simulink model "model_quad_nl_mpc_nl"  (R2021b)
settings: Solver=FixedStepAuto  StartTime=0.0  StopTime=10  FixedStep=.01  MaxStep=.1  MinStep=.005  RelTol=1e-3
values from neighbouring files (symbols this model uses):
  Abody = pi*Rbody^2    (= 0.0314159265359)    [model_quad_init.m]    (also in nlStateFcn.m = 0.0314)
  CDbody = 0.75    [model_quad_init.m]    (also in nlStateFcn.m)
  CT = 0.0248    [model_quad_init.m]
  g = 9.81    [model_quad_init.m]    (also in nlStateFcn.m; nlStateFcnTest.m; start_drone.m)
  i0 = 0    [model_quad_init.m]    (also in nlStateFcn.m)
  Ibbperp = .00942    (= 0.00942)    [model_quad_init.m]    (also in nlStateFcn.m; nlStateFcnTest.m)
  Ibbxx = Ibbperp    (= 0.00942)    [model_quad_init.m]    (also in nlStateFcn.m; nlStateFcnTest.m)
  Ibbxz = 0    [model_quad_init.m]    (also in nlStateFcn.m; nlStateFcnTest.m)
  Ibbyy = Ibbperp    (= 0.00942)    [model_quad_init.m]    (also in nlStateFcn.m; nlStateFcnTest.m)
  Ibbzz = .01867    (= 0.01867)    [model_quad_init.m]    (also in nlStateFcn.m; nlStateFcnTest.m)
  Irrperp = Irrpolar/2    (= 0.0001113)    [model_quad_init.m]    (also in nlStateFcn.m; nlStateFcnTest.m)
  Irrpolar = .0002226    (= 0.0002226)    [model_quad_init.m]
  Kv = 130    [model_quad_init.m]    (also in nlStateFcn.m)
  mb = mb/m_tot    (= 0.760306807287)    [model_quad_init.m]    (also in nlStateFcn.m; nlStateFcnTest.m)
  mr = mr/m_tot    (= 0.0599232981783)    [model_quad_init.m]    (also in nlStateFcn.m; nlStateFcnTest.m)
  R_arms = .45/2    (= 0.225)    [model_quad_init.m]    (also in nlStateFcn.m; nlStateFcnTest.m)
  R_rotor = .125    (= 0.125)    [model_quad_init.m]    (also in nlStateFcn.m)
  rho = 1.225    [model_quad_init.m]    (also in nlStateFcn.m)
  rotorAero = load('loopQuadBET_fromTheBook.mat','C_T','C_H','C_M','C_Q','mu_z_loops','mu_x_loops')    [model_quad_init.m]    (also in nlStateFcn.m)
  Rwinding = 0.56    [model_quad_init.m]
  spin_dir = [1 -1 1 -1]    [model_quad_init.m]    (also in nlStateFcn.m = [1,-1,1,-1])
  Vmax = 4*3.7    (= 14.8)    [model_quad_init.m]
  z_rotors = 0    [model_quad_init.m]    (also in nlStateFcn.m; nlStateFcnTest.m)
undefined symbols (not defined in the file or in its folder): R_RB
libraries: dspmathops x1, mpclib x1
(part 1 of 2)
settings Model: Creator=Elena  LastModifiedBy=Elena

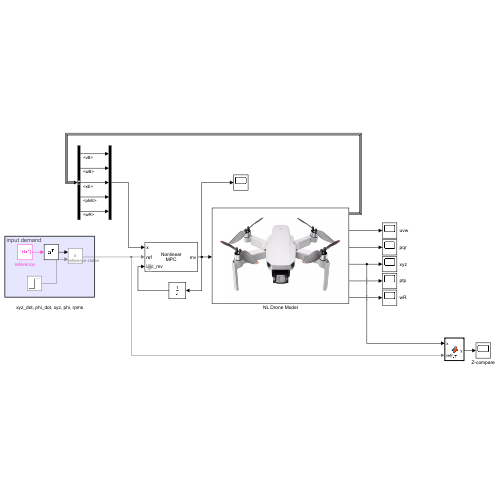
[thumbnail: Simulink's stored preview of the top-level diagram]
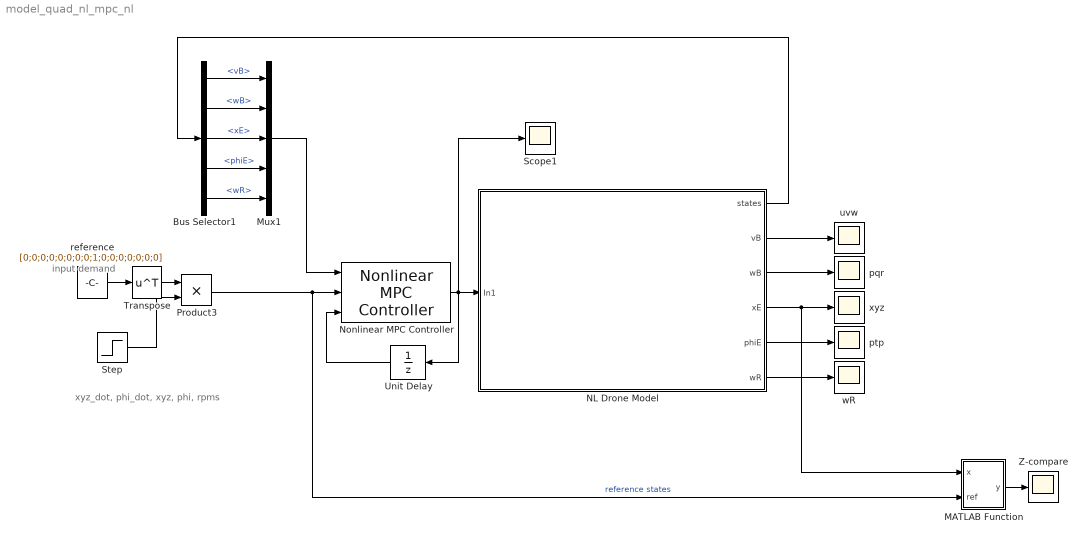
== system model_quad_nl_mpc_nl ==
  note: input demand
  note: xyz_dot, phi_dot, xyz, phi, rpms
  Bus Selector1 : BusSelector  OutputSignals=vB,wB,xE,phiE,wR
  MATLAB Function : MATLAB Function  TreatAsAtomicUnit=on
  Mux1 : Mux  Inputs=5
  NL Drone Model : Subsystem
      mask Display: image('drone_model.png'); % Use "Edit Image" on toolstrip to change.
  Nonlinear MPC Controller : mpclib/Nonlinear MPC Controller  nlmpcobj=nlobj  UseObjectTs=on  UseMEX=off  md_enabled=off  mvtarget_enabled=off  param_enabled=off  cost_enabled=off  mvseq_enabled=off  stateseq_enabled=off  ovseq_enabled=off  slack_enabled=off  status_enabled=off  ov_min=off  ov_max=off  mv_min=off  mv_max=off  mvrate_min=off  mvrate_max=off  state_min=off  state_max=off  ov_weight=off  mv_weight=off  mvrate_weight=off  ecr_weight=off  nlp_initialize=off
  Product3 : Product
  Scope1 : Scope
  Step : Step  SampleTime=0
  Transpose : Math  Operator=transpose  SaturateOnIntegerOverflow=on
  Unit Delay : UnitDelay  SampleTime=-1  HasFrameUpgradeWarning=on
  Z-compare : Scope
  pqr : Scope
  ptp : Scope
  reference : Constant  Value=[0;0;0;0;0;0;0;0;1;0;0;0;0;0;0;0]
  uvw : Scope
  wR : Scope
  xyz : Scope
  wires:
  reference/1 -> Transpose/1
  Step/1 -> Product3/2
  NL Drone Model/4(xE) -> xyz/1, MATLAB Function/1(x)
  Product3/1 -> MATLAB Function/2(ref), Nonlinear MPC Controller/2  "reference states"
  NL Drone Model/1(states) -> Bus Selector1/1
  Bus Selector1/1 -> Mux1/1  "<vB>"
  Bus Selector1/2 -> Mux1/2  "<wB>"
  Bus Selector1/3 -> Mux1/3  "<xE>"
  Bus Selector1/4 -> Mux1/4  "<phiE>"
  Bus Selector1/5 -> Mux1/5  "<wR>"
  Mux1/1 -> Nonlinear MPC Controller/1
  Nonlinear MPC Controller/1 -> Unit Delay/1, NL Drone Model/1(In1), Scope1/1
  MATLAB Function/1(y) -> Z-compare/1
  Unit Delay/1 -> Nonlinear MPC Controller/3
  Transpose/1 -> Product3/1
  NL Drone Model/2(vB) -> uvw/1
  NL Drone Model/3(wB) -> pqr/1
  NL Drone Model/5(phiE) -> ptp/1
  NL Drone Model/6(wR) -> wR/1

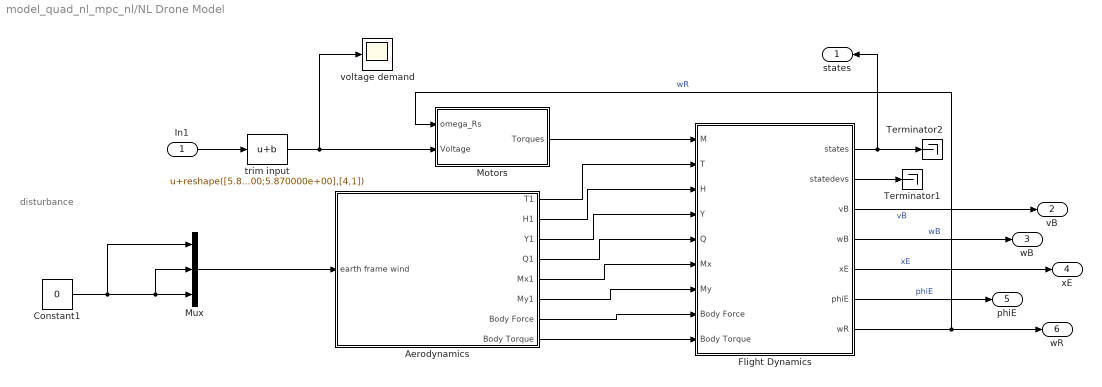
== system model_quad_nl_mpc_nl/NL Drone Model ==
  note: disturbance
  In1 : Inport
  Aerodynamics : Subsystem
  Constant1 : Constant  Value=0
  Flight Dynamics : Subsystem
  Motors : Subsystem
  Mux : Mux  Inputs=3
  Terminator1 : Terminator
  Terminator2 : Terminator
  trim input : Bias  Bias=reshape([5.870000e+00;5.870000e+00;5.870000e+00;5.870000e+00],[4,1])
  voltage demand : Scope
  states : Outport
  vB : Outport  Port=2
  wB : Outport  Port=3
  xE : Outport  Port=4
  phiE : Outport  Port=5
  wR : Outport  Port=6
  wires:
  Aerodynamics/1(T1) -> Flight Dynamics/2(T)
  Flight Dynamics/7(wR) -> wR/1, Motors/1(omega_Rs)  "wR"
  Aerodynamics/6(My1) -> Flight Dynamics/7(My)
  Aerodynamics/2(H1) -> Flight Dynamics/3(H)
  Constant1/1 -> Mux/1, Mux/2, Mux/3
  Aerodynamics/4(Q1) -> Flight Dynamics/5(Q)
  Flight Dynamics/6(phiE) -> phiE/1  "phiE"
  Aerodynamics/7(Body Force) -> Flight Dynamics/8(Body Force)
  Aerodynamics/5(Mx1) -> Flight Dynamics/6(Mx)
  Aerodynamics/8(Body Torque) -> Flight Dynamics/9(Body Torque)
  Flight Dynamics/4(wB) -> wB/1  "wB"
  Flight Dynamics/1(states) -> states/1, Terminator2/1
  Flight Dynamics/2(statedevs) -> Terminator1/1
  Motors/1(Torques) -> Flight Dynamics/1(M)
  Aerodynamics/3(Y1) -> Flight Dynamics/4(Y)
  trim input/1 -> Motors/2(Voltage), voltage demand/1
  In1/1 -> trim input/1
  Mux/1 -> Aerodynamics/1(earth frame wind)
  Flight Dynamics/5(xE) -> xE/1  "xE"
  Flight Dynamics/3(vB) -> vB/1  "vB"

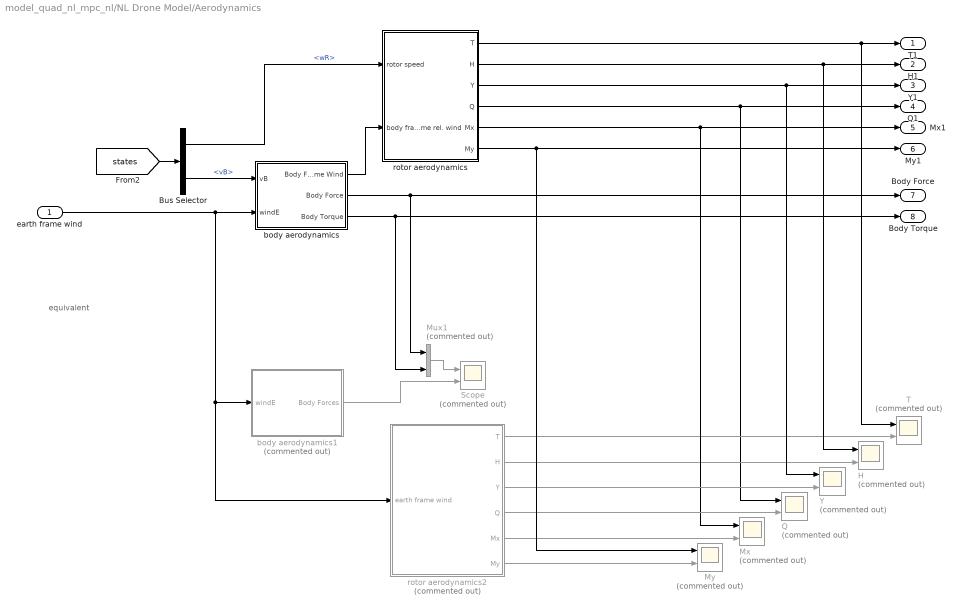
== system model_quad_nl_mpc_nl/NL Drone Model/Aerodynamics ==
  note: equivalent
  earth frame wind : Inport
  Bus Selector : BusSelector  OutputSignals=wR,vB
  H : Scope  Commented=on  NumInputPorts=2
  Mux1 : Mux  Commented=on  Inputs=2
  Mx : Scope  Commented=on  NumInputPorts=2
  My : Scope  Commented=on  NumInputPorts=2
  Q : Scope  Commented=on  NumInputPorts=2
  Scope : Scope  Commented=on  NumInputPorts=2
  T : Scope  Commented=on  NumInputPorts=2
  Y : Scope  Commented=on  NumInputPorts=2
  body aerodynamics : Subsystem
  body aerodynamics1 : Subsystem  Commented=on
  rotor aerodynamics : Subsystem
  rotor aerodynamics2 : Subsystem  Commented=on
  T1 : Outport
  H1 : Outport  Port=2
  Y1 : Outport  Port=3
  Q1 : Outport  Port=4
  Mx1 : Outport  Port=5
  My1 : Outport  Port=6
  Body Force : Outport  Port=7
  Body Torque : Outport  Port=8
  wires:
  rotor aerodynamics/4(Q) -> Q1/1, Q/1
  rotor aerodynamics2/1(T) -> T/2
  earth frame wind/1 -> rotor aerodynamics2/1(earth frame wind), body aerodynamics1/1(windE), body aerodynamics/2(windE)
  Bus Selector/2 -> body aerodynamics/1(vB)  "<vB>"
  rotor aerodynamics2/2(H) -> H/2
  rotor aerodynamics/3(Y) -> Y1/1, Y/1
  rotor aerodynamics/2(H) -> H1/1, H/1
  rotor aerodynamics/5(Mx) -> Mx1/1, Mx/1
  Mux1/1 -> Scope/1
  rotor aerodynamics2/3(Y) -> Y/2
  rotor aerodynamics2/4(Q) -> Q/2
  rotor aerodynamics2/5(Mx) -> Mx/2
  rotor aerodynamics2/6(My) -> My/2
  rotor aerodynamics/6(My) -> My1/1, My/1
  body aerodynamics/1(Body Frame Wind) -> rotor aerodynamics/2(body frame rel. wind)
  body aerodynamics1/1(Body Forces) -> Scope/2
  rotor aerodynamics/1(T) -> T1/1, T/1
  body aerodynamics/3(Body Torque) -> Body Torque/1, Mux1/2
  body aerodynamics/2(Body Force) -> Body Force/1, Mux1/1
  Bus Selector/1 -> rotor aerodynamics/1(rotor speed)  "<wR>"
  [states] -> Bus Selector/1

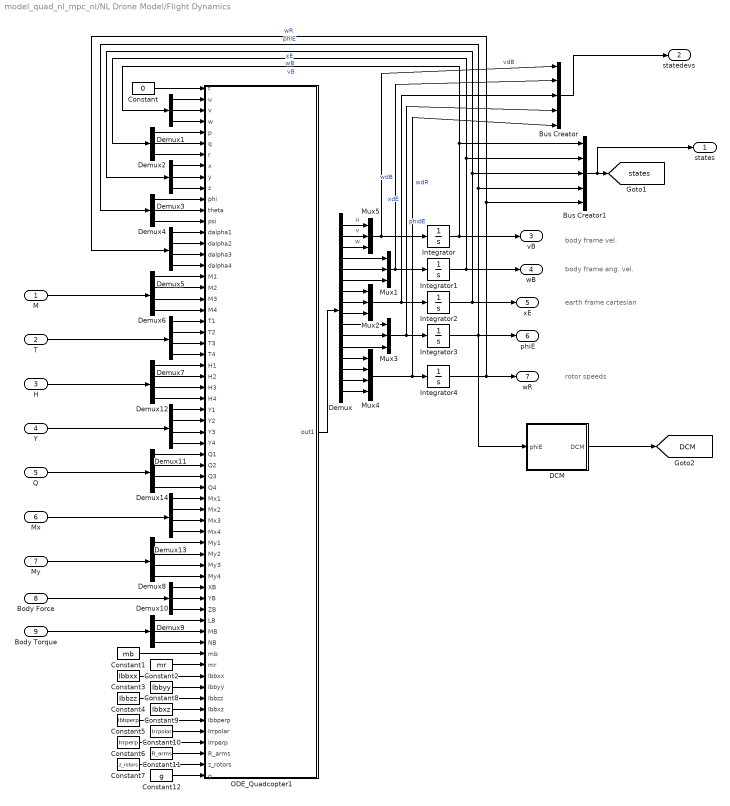
== system model_quad_nl_mpc_nl/NL Drone Model/Flight Dynamics ==
  note: rotor speeds
  note: earth frame cartesian
  note: body frame ang. vel.
  note: body frame vel.
  M : Inport
  T : Inport  Port=2
  H : Inport  Port=3
  Y : Inport  Port=4
  Q : Inport  Port=5
  Mx : Inport  Port=6
  My : Inport  Port=7
  Body Force : Inport  Port=8
  Body Torque : Inport  Port=9
  Bus Creator : BusCreator  Inputs=5
  Bus Creator1 : BusCreator  Inputs=5
  Constant : Constant  Value=0
  Constant1 : Constant  Value=mb
  Constant10 : Constant  Value=Irrpolar
  Constant11 : Constant  Value=R_arms
  Constant12 : Constant  Value=g
  Constant2 : Constant  Value=mr
  Constant3 : Constant  Value=Ibbxx
  Constant4 : Constant  Value=Ibbzz
  Constant5 : Constant  Value=Ibbperp
  Constant6 : Constant  Value=Irrperp
  Constant7 : Constant  Value=z_rotors
  Constant8 : Constant  Value=Ibbyy
  Constant9 : Constant  Value=Ibbxz
  DCM : Subsystem
  Demux : Demux  Outputs=16
  Demux{1..4,9..10} (6 alike) : Demux  Outputs=3
  Demux{5..8,11..14} (8 alike) : Demux
  Integrator{,1..3} (4 alike) : Integrator
  Integrator4 : Integrator  InitialCondition=4386*2*pi/60*[1;1;1;1]
  Mux{1..3,5} (4 alike) : Mux  Inputs=3
  Mux4 : Mux
  ODE_Quadcopter1 : MATLAB Function  TreatAsAtomicUnit=on
  states : Outport
  statedevs : Outport  Port=2
  vB : Outport  Port=3
  wB : Outport  Port=4
  xE : Outport  Port=5
  phiE : Outport  Port=6
  wR : Outport  Port=7
  tag scope: DCM=global, states=global
  wires:
  Body Torque/1 -> Demux10/1
  Body Force/1 -> Demux9/1
  DCM/1(DCM) -> [DCM]
  Bus Creator1/1 -> [states], states/1
  Bus Creator/1 -> statedevs/1
  Integrator3/1 -> DCM/1(phiE), Demux4/1, Bus Creator1/4, phiE/1  "phiE"
  Mux5/1 -> Bus Creator/1, Integrator/1  "vdB"
  Demux/3 -> Mux5/3  "w"
  Demux/2 -> Mux5/2  "v"
  Demux/1 -> Mux5/1  "u"
  Demux5/2 -> ODE_Quadcopter1/15(dalpha2)
  Demux2/1 -> ODE_Quadcopter1/5(p)
  Demux7/3 -> ODE_Quadcopter1/24(T3)
  Demux5/4 -> ODE_Quadcopter1/17(dalpha4)
  Demux3/1 -> ODE_Quadcopter1/8(x)
  Demux2/2 -> ODE_Quadcopter1/6(q)
  M/1 -> Demux6/1
  Demux/5 -> Mux1/2
  Demux4/3 -> ODE_Quadcopter1/13(psi)
  Demux3/2 -> ODE_Quadcopter1/9(y)
  Demux/11 -> Mux3/2
  Demux/16 -> Mux4/4
  Demux1/1 -> ODE_Quadcopter1/2(u)
  Demux6/2 -> ODE_Quadcopter1/19(M2)
  T/1 -> Demux7/1
  Demux/14 -> Mux4/2
  Demux/10 -> Mux3/1
  Integrator1/1 -> Demux2/1, Bus Creator1/2, wB/1  "wB"
  ODE_Quadcopter1/1(out1) -> Demux/1
  Demux6/3 -> ODE_Quadcopter1/20(M3)
  Demux1/2 -> ODE_Quadcopter1/3(v)
  Demux6/4 -> ODE_Quadcopter1/21(M4)
  Demux/9 -> Mux2/3
  Demux/6 -> Mux1/3
  Demux3/3 -> ODE_Quadcopter1/10(z)
  Integrator4/1 -> Demux5/1, Bus Creator1/5, wR/1  "wR"
  Demux/12 -> Mux3/3
  Demux2/3 -> ODE_Quadcopter1/7(r)
  Demux4/1 -> ODE_Quadcopter1/11(phi)
  Demux/13 -> Mux4/1
  Demux7/4 -> ODE_Quadcopter1/25(T4)
  Mux2/1 -> Bus Creator/3, Integrator2/1  "xdE"
  Constant/1 -> ODE_Quadcopter1/1(t)
  Integrator2/1 -> Demux3/1, Bus Creator1/3, xE/1  "xE"
  Demux7/1 -> ODE_Quadcopter1/22(T1)
  Mux1/1 -> Bus Creator/2, Integrator1/1  "wdB"
  Demux6/1 -> ODE_Quadcopter1/18(M1)
  Demux/7 -> Mux2/1
  Demux5/3 -> ODE_Quadcopter1/16(dalpha3)
  Demux/15 -> Mux4/3
  Demux7/2 -> ODE_Quadcopter1/23(T2)
  Demux/8 -> Mux2/2
  My/1 -> Demux8/1
  Demux/4 -> Mux1/1
  Demux4/2 -> ODE_Quadcopter1/12(theta)
  Mux4/1 -> Bus Creator/5, Integrator4/1  "wdR"
  Mux3/1 -> Bus Creator/4, Integrator3/1  "phidE"
  Demux1/3 -> ODE_Quadcopter1/4(w)
  Integrator/1 -> vB/1, Demux1/1, Bus Creator1/1  "vB"
  Demux5/1 -> ODE_Quadcopter1/14(dalpha1)
  Y/1 -> Demux11/1
  H/1 -> Demux12/1
  Q/1 -> Demux14/1
  Mx/1 -> Demux13/1
  Demux11/1 -> ODE_Quadcopter1/30(Y1)
  Demux11/2 -> ODE_Quadcopter1/31(Y2)
  Demux11/3 -> ODE_Quadcopter1/32(Y3)
  Demux11/4 -> ODE_Quadcopter1/33(Y4)
  Demux13/1 -> ODE_Quadcopter1/38(Mx1)
  Demux13/3 -> ODE_Quadcopter1/40(Mx3)
  Demux13/2 -> ODE_Quadcopter1/39(Mx2)
  Demux13/4 -> ODE_Quadcopter1/41(Mx4)
  Demux9/2 -> ODE_Quadcopter1/47(YB)
  Demux9/1 -> ODE_Quadcopter1/46(XB)
  Demux9/3 -> ODE_Quadcopter1/48(ZB)
  Constant2/1 -> ODE_Quadcopter1/53(mr)
  Constant8/1 -> ODE_Quadcopter1/55(Ibbyy)
  Constant9/1 -> ODE_Quadcopter1/57(Ibbxz)
  Constant10/1 -> ODE_Quadcopter1/59(Irrpolar)
  Constant11/1 -> ODE_Quadcopter1/61(R_arms)
  Constant12/1 -> ODE_Quadcopter1/63(g)
  Constant7/1 -> ODE_Quadcopter1/62(z_rotors)
  Constant6/1 -> ODE_Quadcopter1/60(Irrperp)
  Constant5/1 -> ODE_Quadcopter1/58(Ibbperp)
  Constant4/1 -> ODE_Quadcopter1/56(Ibbzz)
  Constant3/1 -> ODE_Quadcopter1/54(Ibbxx)
  Constant1/1 -> ODE_Quadcopter1/52(mb)
  Demux10/3 -> ODE_Quadcopter1/51(NB)
  Demux10/2 -> ODE_Quadcopter1/50(MB)
  Demux10/1 -> ODE_Quadcopter1/49(LB)
  Demux8/4 -> ODE_Quadcopter1/45(My4)
  Demux8/3 -> ODE_Quadcopter1/44(My3)
  Demux8/2 -> ODE_Quadcopter1/43(My2)
  Demux8/1 -> ODE_Quadcopter1/42(My1)
  Demux14/1 -> ODE_Quadcopter1/34(Q1)
  Demux14/2 -> ODE_Quadcopter1/35(Q2)
  Demux14/3 -> ODE_Quadcopter1/36(Q3)
  Demux14/4 -> ODE_Quadcopter1/37(Q4)
  Demux12/1 -> ODE_Quadcopter1/26(H1)
  Demux12/2 -> ODE_Quadcopter1/27(H2)
  Demux12/3 -> ODE_Quadcopter1/28(H3)
  Demux12/4 -> ODE_Quadcopter1/29(H4)

== system model_quad_nl_mpc_nl/NL Drone Model/Motors ==
  note: equivalent
  note: signal logging
  omega_Rs : Inport
  Voltage : Inport  Port=2
  Bus Creator : BusCreator  Inputs=4
  Product : Product
  Saturation : Saturate  UpperLimit=Vmax  LowerLimit=0
  Scope : Scope  Commented=on  NumInputPorts=2
  Terminator : Terminator
  motor_blocks : Subsystem
  motor_function : Subsystem  Commented=on
  voltage : Scope  Commented=on
  Torques : Outport
  wires:
  motor_blocks/1(Qm) -> Scope/1, Torques/1, Product/2, Bus Creator/3  "torque"
  Voltage/1 -> Saturation/1  "Voltage"
  omega_Rs/1 -> motor_function/1(omega_r), motor_blocks/1(omega_r), Bus Creator/1, Product/1  "speed"
  Product/1 -> Bus Creator/2  "power"
  Bus Creator/1 -> Terminator/1  "motors"
  motor_function/1(Qm) -> Scope/2
  Saturation/1 -> motor_function/2(V), voltage/1, motor_blocks/2(V), Bus Creator/4  "voltage"

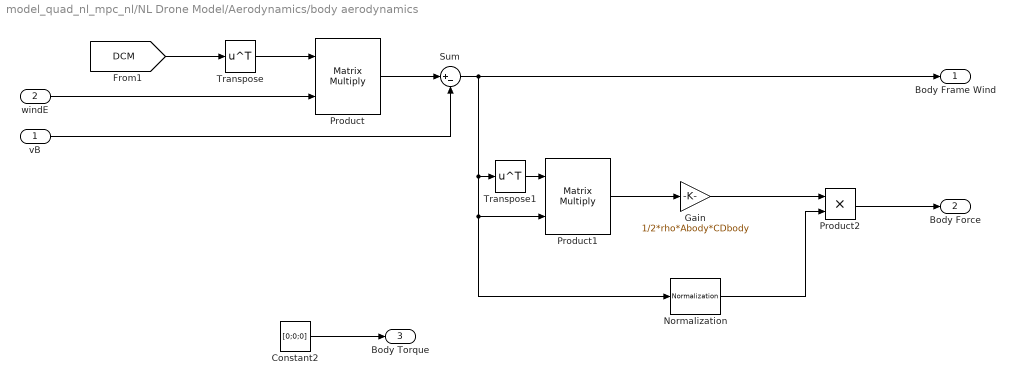
== system model_quad_nl_mpc_nl/NL Drone Model/Aerodynamics/body aerodynamics ==
  vB : Inport
  windE : Inport  Port=2
  Constant2 : Constant  Value=[0;0;0]
  Gain : Gain  Gain=1/2*rho*Abody*CDbody
  Normalization : dspmathops/Normalization  NormType=2-norm  Bias=1e-10  NormOver=Each column  Dimension=1  roundingMode=Floor  overflowMode=off  accumDataTypeStr=Inherit: Same as product output  accumLastDataTypeStr=Inherit: Same as product output  outputDataTypeStr=Inherit: Same as product output  outputMin=[]  outputMax=[]  outputLastDataTypeStr=Inherit: Same as product output
  Product : Product  Multiplication=Matrix(*)
  Product1 : Product  Multiplication=Matrix(*)
  Product2 : Product
  Sum : Sum  Inputs=|+-
  Transpose : Math  Operator=transpose  SaturateOnIntegerOverflow=on
  Transpose1 : Math  Operator=transpose  SaturateOnIntegerOverflow=on
  Body Frame Wind : Outport
  Body Force : Outport  Port=2
  Body Torque : Outport  Port=3
  wires:
  Product2/1 -> Body Force/1
  Constant2/1 -> Body Torque/1
  Transpose/1 -> Product/1
  [DCM] -> Transpose/1
  windE/1 -> Product/2
  Product/1 -> Sum/1
  vB/1 -> Sum/2
  Transpose1/1 -> Product1/1
  Sum/1 -> Body Frame Wind/1, Transpose1/1, Product1/2, Normalization/1
  Product1/1 -> Gain/1
  Gain/1 -> Product2/1
  Normalization/1 -> Product2/2

== system model_quad_nl_mpc_nl/NL Drone Model/Aerodynamics/body aerodynamics1 ==
  windE : Inport
  Bus Selector : BusSelector  OutputSignals=phiE,vB
  Constant : Constant  Value=Abody
  Constant1 : Constant  Value=CDbody
  Constant2 : Constant  Value=rho
  Demux : Demux  Outputs=3
  Demux1 : Demux  Outputs=3
  Demux2 : Demux  Outputs=3
  MATLAB Function : MATLAB Function  TreatAsAtomicUnit=on
  Body Forces : Outport
  wires:
  MATLAB Function/1(FB) -> Body Forces/1
  Constant/1 -> MATLAB Function/1(A_body)
  Constant1/1 -> MATLAB Function/2(C_Dbody)
  [states] -> Bus Selector/1
  Demux/1 -> MATLAB Function/3(phi)
  Demux/2 -> MATLAB Function/6(theta)
  Demux/3 -> MATLAB Function/4(psi)
  Bus Selector/1 -> Demux/1  "<phiE>"
  windE/1 -> Demux1/1
  Demux1/1 -> MATLAB Function/10(w_xE)
  Demux1/2 -> MATLAB Function/11(w_yE)
  Demux1/3 -> MATLAB Function/12(w_zE)
  Constant2/1 -> MATLAB Function/5(rho)
  Demux2/1 -> MATLAB Function/7(u)
  Demux2/2 -> MATLAB Function/8(v)
  Demux2/3 -> MATLAB Function/9(w)
  Bus Selector/2 -> Demux2/1  "<vB>"

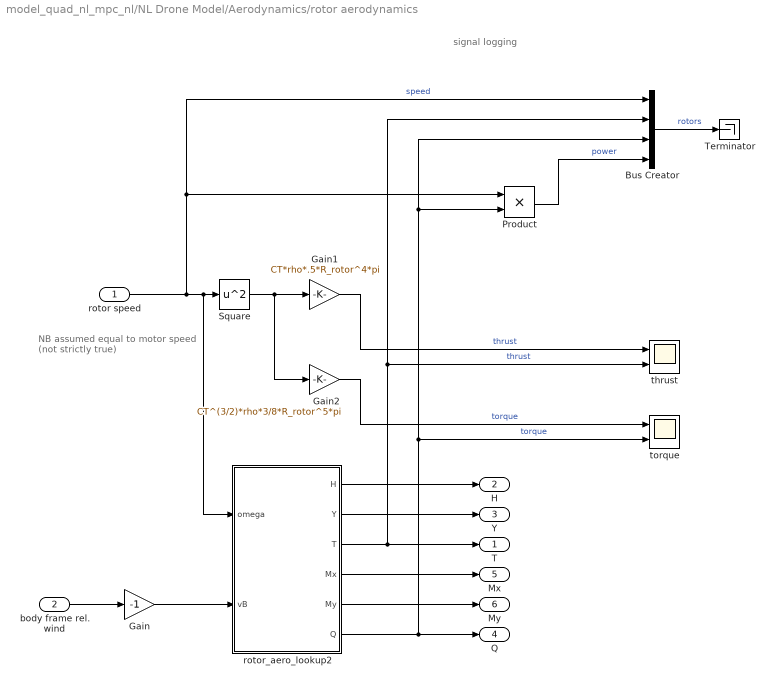
== system model_quad_nl_mpc_nl/NL Drone Model/Aerodynamics/rotor aerodynamics ==
  note: signal logging
  note: NB assumed equal to motor speed
      | (not strictly true)
  rotor speed : Inport
  body frame rel. wind : Inport  Port=2
  Bus Creator : BusCreator  Inputs=4
  Gain : Gain  Gain=-1
  Gain1 : Gain  Gain=CT*rho*.5*R_rotor^4*pi
  Gain2 : Gain  Gain=CT^(3/2)*rho*3/8*R_rotor^5*pi
  Product : Product
  Square : Math  Operator=square  SaturateOnIntegerOverflow=on
  Terminator : Terminator
  rotor_aero_lookup2 : Subsystem  TreatAsAtomicUnit=on
  thrust : Scope  NumInputPorts=2
  torque : Scope  NumInputPorts=2
  T : Outport
  H : Outport  Port=2
  Y : Outport  Port=3
  Q : Outport  Port=4
  Mx : Outport  Port=5
  My : Outport  Port=6
  wires:
  Square/1 -> Gain1/1, Gain2/1
  rotor speed/1 -> rotor_aero_lookup2/1(omega), Square/1, Product/1, Bus Creator/1  "speed"
  rotor_aero_lookup2/3(T) -> T/1, Bus Creator/2, thrust/2  "thrust"
  Product/1 -> Bus Creator/4  "power"
  Bus Creator/1 -> Terminator/1  "rotors"
  body frame rel. wind/1 -> Gain/1
  rotor_aero_lookup2/6(Q) -> Q/1, Product/2, Bus Creator/3, torque/2  "torque"
  Gain1/1 -> thrust/1  "thrust"
  Gain2/1 -> torque/1  "torque"
  rotor_aero_lookup2/1(H) -> H/1
  rotor_aero_lookup2/2(Y) -> Y/1
  rotor_aero_lookup2/5(My) -> My/1
  rotor_aero_lookup2/4(Mx) -> Mx/1
  Gain/1 -> rotor_aero_lookup2/2(vB)

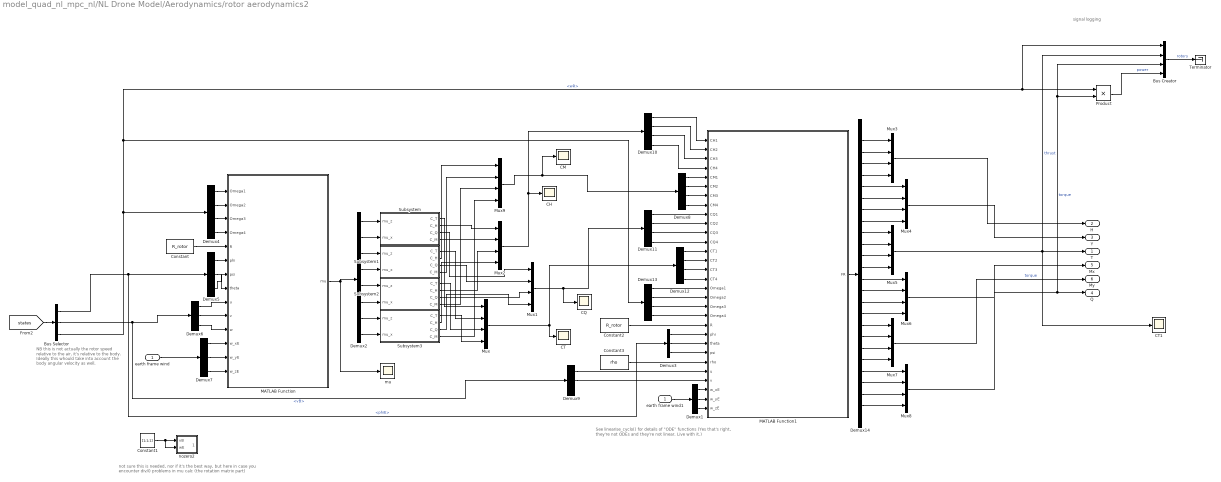
== system model_quad_nl_mpc_nl/NL Drone Model/Aerodynamics/rotor aerodynamics2 ==
  note: not sure this is needed, nor if it's the best way, but here in case you
      | encounter div/0 problems in mu calc (the rotation matrix part)
  note: signal logging
  note: NB this is not actually the rotor speed
      | relative to the air, it's relative to the body.
      | Ideally this whould take into account the
      | body angular velocity as well.
  note: See linearise_cyclo() for details of "ODE" functions
      | (Yes that's right, they're not ODEs and they're not linear. Live with it.)
  earth frame wind : Inport
  Bus Creator : BusCreator  Inputs=4
  Bus Selector : BusSelector  OutputSignals=phiE,vB,wR
  CH : Scope
  CM : Scope
  CQ : Scope
  CT : Scope
  CT1 : Scope
  Constant : Constant  Value=R_rotor
  Constant1 : Constant  Value=[1;1;1]
  Constant2 : Constant  Value=R_rotor
  Constant3 : Constant  Value=rho
  Demux{1,3,5..7,9} (6 alike) : Demux  Outputs=3
  Demux{4,8,10..13} (6 alike) : Demux
  Demux14 : Demux  Outputs=24
  Demux2 : Demux  Outputs=8
  MATLAB Function : MATLAB Function  TreatAsAtomicUnit=on
  MATLAB Function1 : MATLAB Function  TreatAsAtomicUnit=on
  Mux{,1..9} (10 alike) : Mux
  Product : Product
  Subsystem : Subsystem
  Subsystem1 : Subsystem
  Subsystem2 : Subsystem
  Subsystem3 : Subsystem
  Terminator : Terminator
  earth frame wind1 : InportShadow
  mu : Scope
  nozero2 : MATLAB Function  TreatAsAtomicUnit=on
  T : Outport
  H : Outport  Port=2
  Y : Outport  Port=3
  Q : Outport  Port=4
  Mx : Outport  Port=5
  My : Outport  Port=6
  wires:
  Demux9/2 -> MATLAB Function1/27(v)
  Demux9/1 -> MATLAB Function1/26(u)
  Demux3/3 -> MATLAB Function1/24(psi)
  Demux3/2 -> MATLAB Function1/23(theta)
  Demux3/1 -> MATLAB Function1/22(phi)
  Mux9/1 -> Demux8/1, CM/1
  Demux8/4 -> MATLAB Function1/8(CM4)
  Demux8/3 -> MATLAB Function1/7(CM3)
  Demux8/2 -> MATLAB Function1/6(CM2)
  Demux8/1 -> MATLAB Function1/5(CM1)
  earth frame wind1/1 -> Demux1/1
  Demux1/3 -> MATLAB Function1/30(w_zE)
  Demux1/2 -> MATLAB Function1/29(w_yE)
  Demux1/1 -> MATLAB Function1/28(w_xE)
  Subsystem3/4(C_M) -> Mux9/4
  Subsystem2/4(C_M) -> Mux9/3
  Subsystem1/4(C_M) -> Mux9/2
  Subsystem/4(C_M) -> Mux9/1
  Subsystem/3(C_Q) -> Mux1/1
  Subsystem1/3(C_Q) -> Mux1/2
  Subsystem2/3(C_Q) -> Mux1/3
  Subsystem3/3(C_Q) -> Mux1/4
  Subsystem/2(C_H) -> Mux2/1
  Subsystem1/2(C_H) -> Mux2/2
  Subsystem2/2(C_H) -> Mux2/3
  Subsystem3/2(C_H) -> Mux2/4
  Subsystem/1(C_T) -> Mux/1
  Subsystem1/1(C_T) -> Mux/2
  Subsystem2/1(C_T) -> Mux/3
  Subsystem3/1(C_T) -> Mux/4
  Demux4/4 -> MATLAB Function/4(Omega4)
  Demux4/3 -> MATLAB Function/3(Omega3)
  Demux4/2 -> MATLAB Function/2(Omega2)
  Demux4/1 -> MATLAB Function/1(Omega1)
  Bus Selector/2 -> Demux9/1, Demux6/1  "<vB>"
  [states] -> Bus Selector/1
  Bus Selector/1 -> Demux3/1, Demux5/1  "<phiE>"
  Bus Selector/3 -> Demux4/1, Product/1, Bus Creator/1, Demux13/1  "<wR>"
  Demux14/24 -> Mux8/4
  Demux14/23 -> Mux8/3
  Demux14/22 -> Mux8/2
  Demux14/21 -> Mux8/1
  Demux14/20 -> Mux7/4
  Demux14/19 -> Mux7/3
  Demux14/18 -> Mux7/2
  Demux14/17 -> Mux7/1
  Demux14/16 -> Mux6/4
  Demux14/15 -> Mux6/3
  Demux14/14 -> Mux6/2
  Demux14/13 -> Mux6/1
  Demux14/12 -> Mux5/4
  Demux14/11 -> Mux5/3
  Demux14/10 -> Mux5/2
  Demux14/9 -> Mux5/1
  Demux14/8 -> Mux4/4
  Demux14/7 -> Mux4/3
  Demux14/6 -> Mux4/2
  Demux14/5 -> Mux4/1
  Demux14/4 -> Mux3/4
  Demux14/3 -> Mux3/3
  Demux14/2 -> Mux3/2
  Demux14/1 -> Mux3/1
  MATLAB Function1/1(FR) -> Demux14/1
  Mux2/1 -> Demux10/1, CH/1
  Mux1/1 -> Demux11/1, CQ/1
  Mux/1 -> CT/1, Demux12/1
  Demux2/8 -> Subsystem3/2(mu_x)
  Demux2/7 -> Subsystem3/1(mu_z)
  Demux2/6 -> Subsystem2/2(mu_x)
  Demux2/5 -> Subsystem2/1(mu_z)
  Demux2/4 -> Subsystem1/2(mu_x)
  Demux2/3 -> Subsystem1/1(mu_z)
  Demux2/2 -> Subsystem/2(mu_x)
  Demux2/1 -> Subsystem/1(mu_z)
  Constant3/1 -> MATLAB Function1/25(rho)
  Constant2/1 -> MATLAB Function1/21(R)
  Demux13/4 -> MATLAB Function1/20(Omega4)
  Demux13/3 -> MATLAB Function1/19(Omega3)
  Demux13/2 -> MATLAB Function1/18(Omega2)
  Demux13/1 -> MATLAB Function1/17(Omega1)
  Demux12/4 -> MATLAB Function1/16(CT4)
  Demux12/3 -> MATLAB Function1/15(CT3)
  Demux12/2 -> MATLAB Function1/14(CT2)
  Demux12/1 -> MATLAB Function1/13(CT1)
  Demux11/4 -> MATLAB Function1/12(CQ4)
  Demux11/3 -> MATLAB Function1/11(CQ3)
  Demux11/2 -> MATLAB Function1/10(CQ2)
  Demux11/1 -> MATLAB Function1/9(CQ1)
  Demux10/4 -> MATLAB Function1/4(CH4)
  Demux10/3 -> MATLAB Function1/3(CH3)
  Demux10/2 -> MATLAB Function1/2(CH2)
  Demux10/1 -> MATLAB Function1/1(CH1)
  Demux7/3 -> MATLAB Function/14(w_zE)
  Demux7/2 -> MATLAB Function/13(w_yE)
  Demux7/1 -> MATLAB Function/12(w_xE)
  Demux6/3 -> MATLAB Function/11(w)
  Demux6/2 -> MATLAB Function/10(v)
  Demux6/1 -> MATLAB Function/9(u)
  Demux5/3 -> MATLAB Function/7(psi)
  Demux5/1 -> MATLAB Function/6(phi)
  Demux5/2 -> MATLAB Function/8(theta)
  Constant/1 -> MATLAB Function/5(R)
  MATLAB Function/1(mu) -> mu/1, Demux2/1
  Mux6/1 -> Mx/1
  Mux8/1 -> Q/1, Product/2, Bus Creator/3  "torque"
  Mux4/1 -> Y/1
  Mux3/1 -> H/1
  Mux7/1 -> My/1  "torque"
  Bus Creator/1 -> Terminator/1  "rotors"
  Product/1 -> Bus Creator/4  "power"
  Mux5/1 -> T/1, Bus Creator/2, CT1/1  "thrust"
  earth frame wind/1 -> Demux7/1
  Constant1/1 -> nozero2/2(wE), nozero2/1(vB)

== system model_quad_nl_mpc_nl/NL Drone Model/Flight Dynamics/DCM ==
  phiE : Inport
  Demux9 : Demux  Outputs=3
  MATLAB Function : MATLAB Function  TreatAsAtomicUnit=on
  DCM : Outport
  wires:
  MATLAB Function/1(DCM) -> DCM/1
  Demux9/2 -> MATLAB Function/2(theta)
  phiE/1 -> Demux9/1
  Demux9/3 -> MATLAB Function/3(psi)
  Demux9/1 -> MATLAB Function/1(phi)

== system model_quad_nl_mpc_nl/NL Drone Model/Motors/motor_blocks ==
  note: assume ESC can't brake
  note: Qm=( (v-omega/Kv)/R - i0)/Kv
  omega_r : Inport
  V : Inport  Port=2
  Constant : Constant  Value=Kv
  Constant1 : Constant  Value=Rwinding
  Constant2 : Constant  Value=i0
  Divide : Product  Inputs=*/
  Divide1 : Product  Inputs=*/
  Divide2 : Product  Inputs=*/
  Saturation : Saturate  UpperLimit=inf  LowerLimit=0
  Sum : Sum  Inputs=|+-
  Sum1 : Sum  Inputs=|+-
  Qm : Outport
  wires:
  Divide2/1 -> Saturation/1
  Sum1/1 -> Divide2/1
  Constant2/1 -> Sum1/2
  Divide1/1 -> Sum1/1  "i"
  Constant1/1 -> Divide1/2
  Sum/1 -> Divide1/1
  Divide/1 -> Sum/2
  Constant/1 -> Divide/2, Divide2/2
  omega_r/1 -> Divide/1
  V/1 -> Sum/1
  Saturation/1 -> Qm/1

== system model_quad_nl_mpc_nl/NL Drone Model/Motors/motor_function ==
  note: assume ESC can't brake
  omega_r : Inport
  V : Inport  Port=2
  Constant : Constant  Value=Kv
  Constant1 : Constant  Value=Rwinding
  Demux : Demux
  Demux1 : Demux
  MATLAB Function : MATLAB Function  TreatAsAtomicUnit=on
  Saturation1 : Saturate  UpperLimit=inf  LowerLimit=0
  Qm : Outport
  wires:
  Demux1/1 -> MATLAB Function/7(V1)
  Constant/1 -> MATLAB Function/1(K_v)
  Demux/1 -> MATLAB Function/2(Omega1)
  Demux/3 -> MATLAB Function/4(Omega3)
  Demux/2 -> MATLAB Function/3(Omega2)
  omega_r/1 -> Demux/1
  Demux/4 -> MATLAB Function/5(Omega4)
  Constant1/1 -> MATLAB Function/6(R_winding)
  Demux1/2 -> MATLAB Function/8(V2)
  Demux1/4 -> MATLAB Function/10(V4)
  Demux1/3 -> MATLAB Function/9(V3)
  MATLAB Function/1(M) -> Saturation1/1
  Saturation1/1 -> Qm/1
  V/1 -> Demux1/1

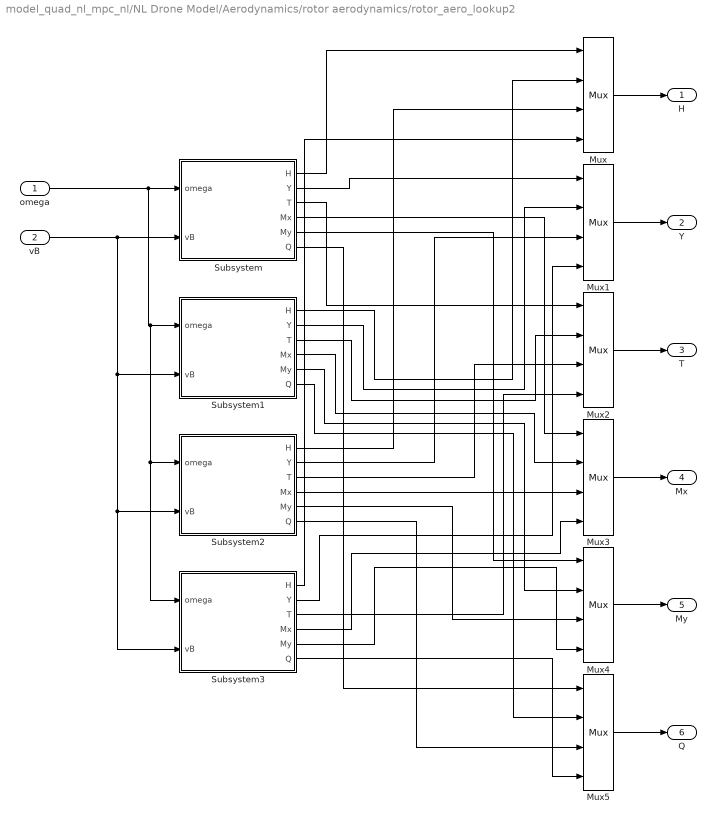
== system model_quad_nl_mpc_nl/NL Drone Model/Aerodynamics/rotor aerodynamics/rotor_aero_lookup2 ==
  omega : Inport
  vB : Inport  Port=2
  Mux{,1..5} (6 alike) : Mux
  Subsystem : Subsystem  mask{motor_num=1}
      mask prompts: motor_num "motor number"
      mask TypeOptions motor_num: 1 | 2 | 3 | 4
      mask Display: disp(get_param(gcb,'motor_num'));
  Subsystem1 : Subsystem  mask{motor_num=2}
      mask prompts: motor_num "motor number"
      mask TypeOptions motor_num: 1 | 2 | 3 | 4
      mask Display: disp(get_param(gcb,'motor_num'));
  Subsystem2 : Subsystem  mask{motor_num=3}
      mask prompts: motor_num "motor number"
      mask TypeOptions motor_num: 1 | 2 | 3 | 4
      mask Display: disp(get_param(gcb,'motor_num'));
  Subsystem3 : Subsystem  mask{motor_num=4}
      mask prompts: motor_num "motor number"
      mask TypeOptions motor_num: 1 | 2 | 3 | 4
      mask Display: disp(get_param(gcb,'motor_num'));
  H : Outport
  Y : Outport  Port=2
  T : Outport  Port=3
  Mx : Outport  Port=4
  My : Outport  Port=5
  Q : Outport  Port=6
  wires:
  omega/1 -> Subsystem1/1(omega), Subsystem3/1(omega), Subsystem2/1(omega), Subsystem/1(omega)
  vB/1 -> Subsystem1/2(vB), Subsystem3/2(vB), Subsystem2/2(vB), Subsystem/2(vB)
  Subsystem/1(H) -> Mux/1
  Subsystem/2(Y) -> Mux1/1
  Mux/1 -> H/1
  Subsystem1/1(H) -> Mux/2
  Subsystem2/1(H) -> Mux/3
  Subsystem3/1(H) -> Mux/4
  Mux1/1 -> Y/1
  Subsystem1/2(Y) -> Mux1/2
  Subsystem2/2(Y) -> Mux1/3
  Subsystem3/2(Y) -> Mux1/4
  Subsystem/3(T) -> Mux2/1
  Subsystem1/3(T) -> Mux2/2
  Subsystem2/3(T) -> Mux2/3
  Subsystem3/3(T) -> Mux2/4
  Mux2/1 -> T/1
  Subsystem/4(Mx) -> Mux3/1
  Subsystem1/4(Mx) -> Mux3/2
  Subsystem2/4(Mx) -> Mux3/3
  Subsystem3/4(Mx) -> Mux3/4
  Subsystem/5(My) -> Mux4/1
  Subsystem1/5(My) -> Mux4/2
  Subsystem2/5(My) -> Mux4/3
  Subsystem3/5(My) -> Mux4/4
  Subsystem/6(Q) -> Mux5/1
  Subsystem1/6(Q) -> Mux5/2
  Subsystem2/6(Q) -> Mux5/3
  Subsystem3/6(Q) -> Mux5/4
  Mux3/1 -> Mx/1
  Mux4/1 -> My/1
  Mux5/1 -> Q/1

== system model_quad_nl_mpc_nl/NL Drone Model/Aerodynamics/rotor aerodynamics2/Subsystem ==
  mu_z : Inport
  mu_x : Inport  Port=2
  C_H1 : Lookup_n-D  BreakpointsForDimension1=rotorAero.mu_x_loops  BreakpointsForDimension2=rotorAero.mu_z_loops  Table=rotorAero.C_H  InternalRulePriority=Speed  RndMeth=Simplest  InputSameDT=on
      settings: InputPortMap=u0,u1
  C_M1 : Lookup_n-D  BreakpointsForDimension1=rotorAero.mu_x_loops  BreakpointsForDimension2=rotorAero.mu_z_loops  Table=rotorAero.C_M  InternalRulePriority=Speed  RndMeth=Simplest  InputSameDT=on
      settings: InputPortMap=u0,u1
  C_Q1 : Lookup_n-D  BreakpointsForDimension1=rotorAero.mu_x_loops  BreakpointsForDimension2=rotorAero.mu_z_loops  Table=rotorAero.C_Q  InternalRulePriority=Speed  RndMeth=Simplest  InputSameDT=on
      settings: InputPortMap=u0,u1
  C_T 1 : Lookup_n-D  BreakpointsForDimension1=rotorAero.mu_x_loops  BreakpointsForDimension2=rotorAero.mu_z_loops  Table=rotorAero.C_T  InternalRulePriority=Speed  RndMeth=Simplest  InputSameDT=on
      settings: InputPortMap=u0,u1
  C_T : Outport
  C_H : Outport  Port=2
  C_Q : Outport  Port=3
  C_M : Outport  Port=4
  wires:
  C_M1/1 -> C_M/1
  C_Q1/1 -> C_Q/1
  C_T 1/1 -> C_T/1
  C_H1/1 -> C_H/1
  mu_z/1 -> C_H1/2, C_Q1/2, C_M1/2, C_T 1/2
  mu_x/1 -> C_H1/1, C_Q1/1, C_M1/1, C_T 1/1

== system model_quad_nl_mpc_nl/NL Drone Model/Aerodynamics/rotor aerodynamics2/Subsystem1 ==
  mu_z : Inport
  mu_x : Inport  Port=2
  C_H1 : Lookup_n-D  BreakpointsForDimension1=rotorAero.mu_x_loops  BreakpointsForDimension2=rotorAero.mu_z_loops  Table=rotorAero.C_H  InternalRulePriority=Speed  RndMeth=Simplest  InputSameDT=on
      settings: InputPortMap=u0,u1
  C_M1 : Lookup_n-D  BreakpointsForDimension1=rotorAero.mu_x_loops  BreakpointsForDimension2=rotorAero.mu_z_loops  Table=rotorAero.C_M  InternalRulePriority=Speed  RndMeth=Simplest  InputSameDT=on
      settings: InputPortMap=u0,u1
  C_Q1 : Lookup_n-D  BreakpointsForDimension1=rotorAero.mu_x_loops  BreakpointsForDimension2=rotorAero.mu_z_loops  Table=rotorAero.C_Q  InternalRulePriority=Speed  RndMeth=Simplest  InputSameDT=on
      settings: InputPortMap=u0,u1
  C_T 1 : Lookup_n-D  BreakpointsForDimension1=rotorAero.mu_x_loops  BreakpointsForDimension2=rotorAero.mu_z_loops  Table=rotorAero.C_T  InternalRulePriority=Speed  RndMeth=Simplest  InputSameDT=on
      settings: InputPortMap=u0,u1
  C_T : Outport
  C_H : Outport  Port=2
  C_Q : Outport  Port=3
  C_M : Outport  Port=4
  wires:
  mu_x/1 -> C_T 1/1, C_M1/1, C_Q1/1, C_H1/1
  mu_z/1 -> C_T 1/2, C_M1/2, C_Q1/2, C_H1/2
  C_H1/1 -> C_H/1
  C_T 1/1 -> C_T/1
  C_Q1/1 -> C_Q/1
  C_M1/1 -> C_M/1

== system model_quad_nl_mpc_nl/NL Drone Model/Aerodynamics/rotor aerodynamics2/Subsystem2 ==
  mu_z : Inport
  mu_x : Inport  Port=2
  C_H1 : Lookup_n-D  BreakpointsForDimension1=rotorAero.mu_x_loops  BreakpointsForDimension2=rotorAero.mu_z_loops  Table=rotorAero.C_H  InternalRulePriority=Speed  RndMeth=Simplest  InputSameDT=on
      settings: InputPortMap=u0,u1
  C_M1 : Lookup_n-D  BreakpointsForDimension1=rotorAero.mu_x_loops  BreakpointsForDimension2=rotorAero.mu_z_loops  Table=rotorAero.C_M  InternalRulePriority=Speed  RndMeth=Simplest  InputSameDT=on
      settings: InputPortMap=u0,u1
  C_Q1 : Lookup_n-D  BreakpointsForDimension1=rotorAero.mu_x_loops  BreakpointsForDimension2=rotorAero.mu_z_loops  Table=rotorAero.C_Q  InternalRulePriority=Speed  RndMeth=Simplest  InputSameDT=on
      settings: InputPortMap=u0,u1
  C_T 1 : Lookup_n-D  BreakpointsForDimension1=rotorAero.mu_x_loops  BreakpointsForDimension2=rotorAero.mu_z_loops  Table=rotorAero.C_T  InternalRulePriority=Speed  RndMeth=Simplest  InputSameDT=on
      settings: InputPortMap=u0,u1
  C_T : Outport
  C_H : Outport  Port=2
  C_Q : Outport  Port=3
  C_M : Outport  Port=4
  wires:
  C_M1/1 -> C_M/1
  C_Q1/1 -> C_Q/1
  C_T 1/1 -> C_T/1
  C_H1/1 -> C_H/1
  mu_z/1 -> C_H1/2, C_Q1/2, C_M1/2, C_T 1/2
  mu_x/1 -> C_H1/1, C_Q1/1, C_M1/1, C_T 1/1

== system model_quad_nl_mpc_nl/NL Drone Model/Aerodynamics/rotor aerodynamics2/Subsystem3 ==
  mu_z : Inport
  mu_x : Inport  Port=2
  C_H1 : Lookup_n-D  BreakpointsForDimension1=rotorAero.mu_x_loops  BreakpointsForDimension2=rotorAero.mu_z_loops  Table=rotorAero.C_H  InternalRulePriority=Speed  RndMeth=Simplest  InputSameDT=on
      settings: InputPortMap=u0,u1
  C_M1 : Lookup_n-D  BreakpointsForDimension1=rotorAero.mu_x_loops  BreakpointsForDimension2=rotorAero.mu_z_loops  Table=rotorAero.C_M  InternalRulePriority=Speed  RndMeth=Simplest  InputSameDT=on
      settings: InputPortMap=u0,u1
  C_Q1 : Lookup_n-D  BreakpointsForDimension1=rotorAero.mu_x_loops  BreakpointsForDimension2=rotorAero.mu_z_loops  Table=rotorAero.C_Q  InternalRulePriority=Speed  RndMeth=Simplest  InputSameDT=on
      settings: InputPortMap=u0,u1
  C_T 1 : Lookup_n-D  BreakpointsForDimension1=rotorAero.mu_x_loops  BreakpointsForDimension2=rotorAero.mu_z_loops  Table=rotorAero.C_T  InternalRulePriority=Speed  RndMeth=Simplest  InputSameDT=on
      settings: InputPortMap=u0,u1
  C_T : Outport
  C_H : Outport  Port=2
  C_Q : Outport  Port=3
  C_M : Outport  Port=4
  wires:
  mu_x/1 -> C_T 1/1, C_M1/1, C_Q1/1, C_H1/1
  mu_z/1 -> C_T 1/2, C_M1/2, C_Q1/2, C_H1/2
  C_H1/1 -> C_H/1
  C_T 1/1 -> C_T/1
  C_Q1/1 -> C_Q/1
  C_M1/1 -> C_M/1

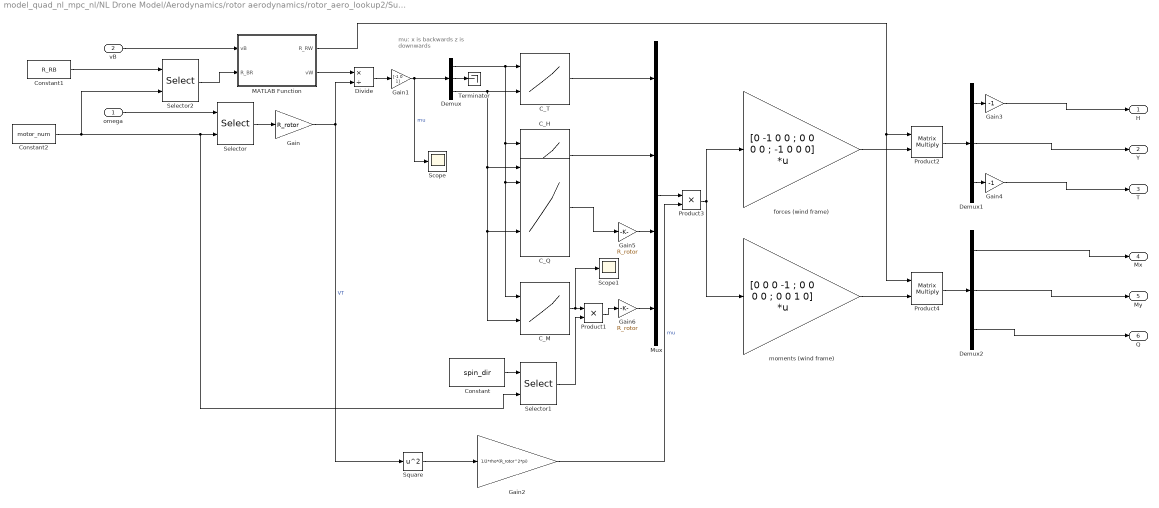
== system model_quad_nl_mpc_nl/NL Drone Model/Aerodynamics/rotor aerodynamics/rotor_aero_lookup2/Subsystem ==
  note: mu:
      | x is backwards
      | z is downwards
  omega : Inport
  vB : Inport  Port=2
  C_H : Lookup_n-D  BreakpointsForDimension1=rotorAero.mu_x_loops  BreakpointsForDimension2=rotorAero.mu_z_loops  Table=rotorAero.C_H  InternalRulePriority=Speed  RndMeth=Simplest  InputSameDT=on
      settings: InputPortMap=u0,u1
  C_M : Lookup_n-D  BreakpointsForDimension1=rotorAero.mu_x_loops  BreakpointsForDimension2=rotorAero.mu_z_loops  Table=rotorAero.C_M  InternalRulePriority=Speed  RndMeth=Simplest  InputSameDT=on
      settings: InputPortMap=u0,u1
  C_Q : Lookup_n-D  BreakpointsForDimension1=rotorAero.mu_x_loops  BreakpointsForDimension2=rotorAero.mu_z_loops  Table=rotorAero.C_Q  InternalRulePriority=Speed  RndMeth=Simplest  InputSameDT=on
      settings: InputPortMap=u0,u1
  "C_T " : Lookup_n-D  BreakpointsForDimension1=rotorAero.mu_x_loops  BreakpointsForDimension2=rotorAero.mu_z_loops  Table=rotorAero.C_T  InternalRulePriority=Speed  RndMeth=Simplest  InputSameDT=on
      settings: InputPortMap=u0,u1
  Constant : Constant  Value=spin_dir
  Constant1 : Constant  Value=R_RB
  Constant2 : Constant  Value=motor_num
  Demux : Demux  Outputs=3
  Demux1 : Demux  Outputs=3
  Demux2 : Demux  Outputs=3
  Divide : Product  Inputs=*/
  Gain : Gain  Gain=R_rotor
  Gain1 : Gain  Gain=[-1 0 1]
  Gain2 : Gain  Gain=1/2*rho*(R_rotor^2*pi)
  Gain3 : Gain  Gain=-1
  Gain4 : Gain  Gain=-1
  Gain5 : Gain  Gain=R_rotor
  Gain6 : Gain  Gain=R_rotor
  MATLAB Function : MATLAB Function  TreatAsAtomicUnit=on
  Mux : Mux
  Product1 : Product
  Product2 : Product  Multiplication=Matrix(*)
  Product3 : Product
  Product4 : Product  Multiplication=Matrix(*)
  Scope : Scope
  Scope1 : Scope
  Selector : Selector  InputPortWidth=4  IndexOptions=Index vector (port)  Indices=[1 3]  OutputSizes=1
  Selector1 : Selector  InputPortWidth=4  IndexOptions=Index vector (port)  Indices=[1 3]  OutputSizes=1
  Selector2 : Selector  NumberOfDimensions=3  InputPortWidth=4  IndexOptions=Select all,Select all,Index vector (port)  Indices=[1 3],1,1  OutputSizes=1,1,1
  Square : Math  Operator=square  SaturateOnIntegerOverflow=on
  Terminator : Terminator
  forces (wind frame) : Gain  Gain=[0 -1 0 0 ; 0 0 0 0 ; -1 0 0 0]  Multiplication=Matrix(K*u) (u vector)
  moments (wind frame) : Gain  Gain=[0 0 0 -1 ; 0 0 0 0 ; 0 0 1 0]  Multiplication=Matrix(K*u) (u vector)
  H : Outport
  Y : Outport  Port=2
  T : Outport  Port=3
  Mx : Outport  Port=4
  My : Outport  Port=5
  Q : Outport  Port=6
  wires:
  Demux/2 -> Terminator/1
  Mux/1 -> Product3/1
  Selector2/1 -> MATLAB Function/2(R_BR)
  Gain4/1 -> T/1
  Demux1/3 -> Gain4/1
  Demux/3 -> "C_T "/2, C_H/2, C_M/2, C_Q/2
  Constant2/1 -> Selector/2, Selector1/2, Selector2/2
  Selector/1 -> Gain/1
  Gain2/1 -> Product3/2  "mu"
  Constant1/1 -> Selector2/1
  Demux1/1 -> Gain3/1
  "C_T "/1 -> Mux/1
  Product4/1 -> Demux2/1
  moments (wind frame)/1 -> Product4/2
  Divide/1 -> Gain1/1
  Square/1 -> Gain2/1
  Demux/1 -> "C_T "/1, C_H/1, C_M/1, C_Q/1
  C_M/1 -> Scope1/1, Product1/1
  C_H/1 -> Mux/2
  Product2/1 -> Demux1/1
  Demux1/2 -> Y/1
  omega/1 -> Selector/1
  Demux2/3 -> Q/1
  vB/1 -> MATLAB Function/1(vB)
  MATLAB Function/1(R_RW) -> Product2/1, Product4/1
  Selector1/1 -> Product1/2
  Demux2/1 -> Mx/1
  MATLAB Function/2(vW) -> Divide/1
  Gain1/1 -> Scope/1, Demux/1  "mu"
  Product3/1 -> moments (wind frame)/1, forces (wind frame)/1
  forces (wind frame)/1 -> Product2/2
  Gain/1 -> Divide/2, Square/1  "VT"
  Demux2/2 -> My/1
  Constant/1 -> Selector1/1
  Gain3/1 -> H/1
  Gain6/1 -> Mux/4
  Gain5/1 -> Mux/3
  Product1/1 -> Gain6/1
  C_Q/1 -> Gain5/1

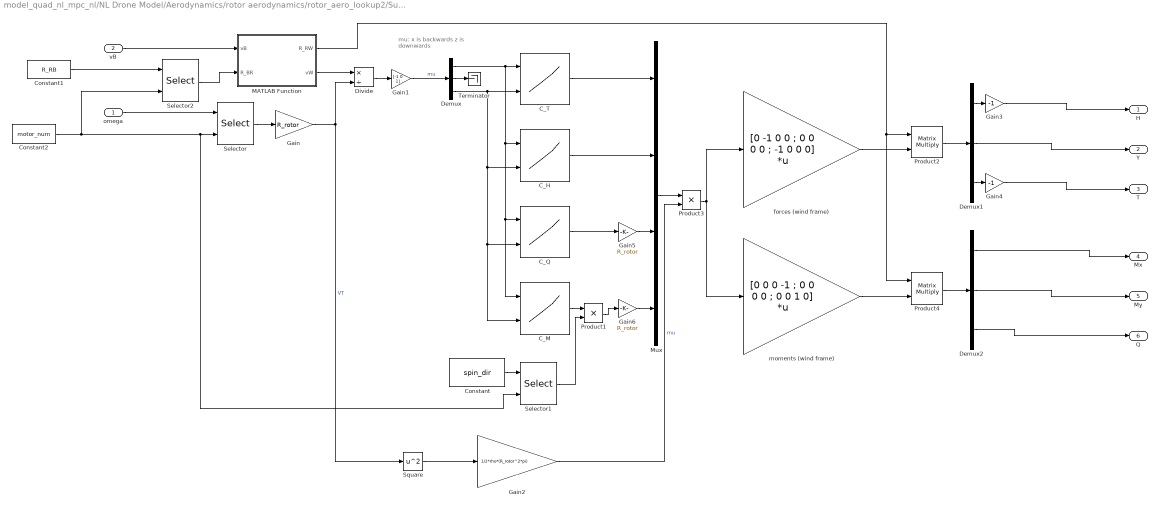
== system model_quad_nl_mpc_nl/NL Drone Model/Aerodynamics/rotor aerodynamics/rotor_aero_lookup2/Subsystem1 ==
  note: mu:
      | x is backwards
      | z is downwards
  omega : Inport
  vB : Inport  Port=2
  C_H : Lookup_n-D  BreakpointsForDimension1=rotorAero.mu_x_loops  BreakpointsForDimension2=rotorAero.mu_z_loops  Table=rotorAero.C_H  InternalRulePriority=Speed  RndMeth=Simplest  InputSameDT=on
      settings: InputPortMap=u0,u1
  C_M : Lookup_n-D  BreakpointsForDimension1=rotorAero.mu_x_loops  BreakpointsForDimension2=rotorAero.mu_z_loops  Table=rotorAero.C_M  InternalRulePriority=Speed  RndMeth=Simplest  InputSameDT=on
      settings: InputPortMap=u0,u1
  C_Q : Lookup_n-D  BreakpointsForDimension1=rotorAero.mu_x_loops  BreakpointsForDimension2=rotorAero.mu_z_loops  Table=rotorAero.C_Q  InternalRulePriority=Speed  RndMeth=Simplest  InputSameDT=on
      settings: InputPortMap=u0,u1
  "C_T " : Lookup_n-D  BreakpointsForDimension1=rotorAero.mu_x_loops  BreakpointsForDimension2=rotorAero.mu_z_loops  Table=rotorAero.C_T  InternalRulePriority=Speed  RndMeth=Simplest  InputSameDT=on
      settings: InputPortMap=u0,u1
  Constant : Constant  Value=spin_dir
  Constant1 : Constant  Value=R_RB
  Constant2 : Constant  Value=motor_num
  Demux : Demux  Outputs=3
  Demux1 : Demux  Outputs=3
  Demux2 : Demux  Outputs=3
  Divide : Product  Inputs=*/
  Gain : Gain  Gain=R_rotor
  Gain1 : Gain  Gain=[-1 0 1]
  Gain2 : Gain  Gain=1/2*rho*(R_rotor^2*pi)
  Gain3 : Gain  Gain=-1
  Gain4 : Gain  Gain=-1
  Gain5 : Gain  Gain=R_rotor
  Gain6 : Gain  Gain=R_rotor
  MATLAB Function : MATLAB Function  TreatAsAtomicUnit=on
  Mux : Mux
  Product1 : Product
  Product2 : Product  Multiplication=Matrix(*)
  Product3 : Product
  Product4 : Product  Multiplication=Matrix(*)
  Selector : Selector  InputPortWidth=4  IndexOptions=Index vector (port)  Indices=[1 3]  OutputSizes=1
  Selector1 : Selector  InputPortWidth=4  IndexOptions=Index vector (port)  Indices=[1 3]  OutputSizes=1
  Selector2 : Selector  NumberOfDimensions=3  InputPortWidth=4  IndexOptions=Select all,Select all,Index vector (port)  Indices=[1 3],1,1  OutputSizes=1,1,1
  Square : Math  Operator=square  SaturateOnIntegerOverflow=on
  Terminator : Terminator
  forces (wind frame) : Gain  Gain=[0 -1 0 0 ; 0 0 0 0 ; -1 0 0 0]  Multiplication=Matrix(K*u) (u vector)
  moments (wind frame) : Gain  Gain=[0 0 0 -1 ; 0 0 0 0 ; 0 0 1 0]  Multiplication=Matrix(K*u) (u vector)
  H : Outport
  Y : Outport  Port=2
  T : Outport  Port=3
  Mx : Outport  Port=4
  My : Outport  Port=5
  Q : Outport  Port=6
  wires:
  C_Q/1 -> Gain5/1
  Product1/1 -> Gain6/1
  Gain5/1 -> Mux/3
  Gain6/1 -> Mux/4
  Gain3/1 -> H/1
  Constant/1 -> Selector1/1
  Demux2/2 -> My/1
  Gain/1 -> Square/1, Divide/2  "VT"
  forces (wind frame)/1 -> Product2/2
  Product3/1 -> forces (wind frame)/1, moments (wind frame)/1
  Gain1/1 -> Demux/1  "mu"
  MATLAB Function/2(vW) -> Divide/1
  Demux2/1 -> Mx/1
  Selector1/1 -> Product1/2
  MATLAB Function/1(R_RW) -> Product4/1, Product2/1
  vB/1 -> MATLAB Function/1(vB)
  Demux2/3 -> Q/1
  omega/1 -> Selector/1
  Demux1/2 -> Y/1
  Product2/1 -> Demux1/1
  C_H/1 -> Mux/2
  C_M/1 -> Product1/1
  Demux/1 -> C_M/1, C_Q/1, C_H/1, "C_T "/1
  Square/1 -> Gain2/1
  Divide/1 -> Gain1/1
  moments (wind frame)/1 -> Product4/2
  Product4/1 -> Demux2/1
  "C_T "/1 -> Mux/1
  Demux1/1 -> Gain3/1
  Constant1/1 -> Selector2/1
  Gain2/1 -> Product3/2  "mu"
  Selector/1 -> Gain/1
  Constant2/1 -> Selector2/2, Selector1/2, Selector/2
  Demux/3 -> C_M/2, C_Q/2, C_H/2, "C_T "/2
  Demux1/3 -> Gain4/1
  Gain4/1 -> T/1
  Selector2/1 -> MATLAB Function/2(R_BR)
  Mux/1 -> Product3/1
  Demux/2 -> Terminator/1

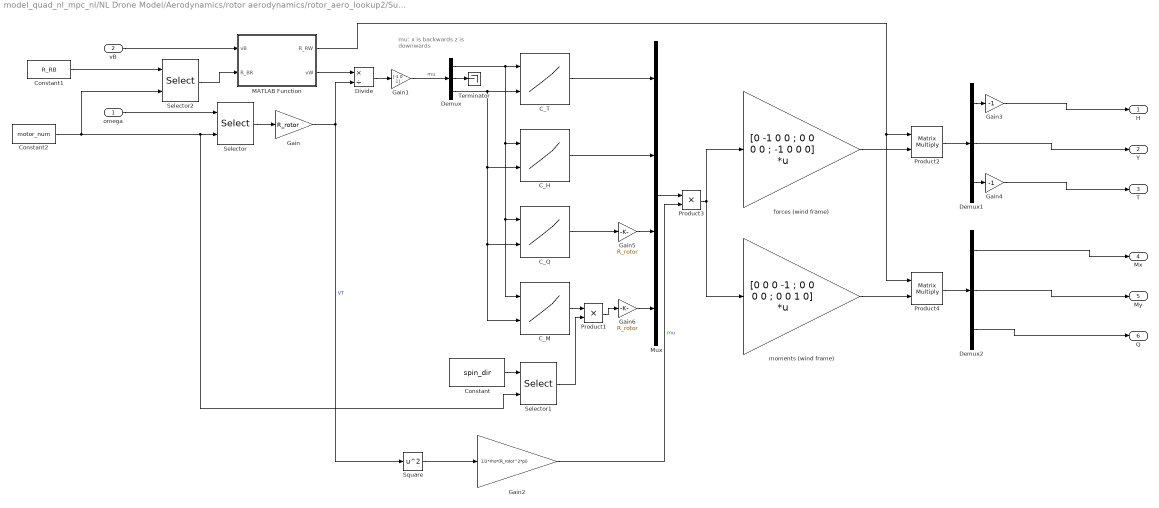
== system model_quad_nl_mpc_nl/NL Drone Model/Aerodynamics/rotor aerodynamics/rotor_aero_lookup2/Subsystem2 ==
  note: mu:
      | x is backwards
      | z is downwards
  omega : Inport
  vB : Inport  Port=2
  C_H : Lookup_n-D  BreakpointsForDimension1=rotorAero.mu_x_loops  BreakpointsForDimension2=rotorAero.mu_z_loops  Table=rotorAero.C_H  InternalRulePriority=Speed  RndMeth=Simplest  InputSameDT=on
      settings: InputPortMap=u0,u1
  C_M : Lookup_n-D  BreakpointsForDimension1=rotorAero.mu_x_loops  BreakpointsForDimension2=rotorAero.mu_z_loops  Table=rotorAero.C_M  InternalRulePriority=Speed  RndMeth=Simplest  InputSameDT=on
      settings: InputPortMap=u0,u1
  C_Q : Lookup_n-D  BreakpointsForDimension1=rotorAero.mu_x_loops  BreakpointsForDimension2=rotorAero.mu_z_loops  Table=rotorAero.C_Q  InternalRulePriority=Speed  RndMeth=Simplest  InputSameDT=on
      settings: InputPortMap=u0,u1
  "C_T " : Lookup_n-D  BreakpointsForDimension1=rotorAero.mu_x_loops  BreakpointsForDimension2=rotorAero.mu_z_loops  Table=rotorAero.C_T  InternalRulePriority=Speed  RndMeth=Simplest  InputSameDT=on
      settings: InputPortMap=u0,u1
  Constant : Constant  Value=spin_dir
  Constant1 : Constant  Value=R_RB
  Constant2 : Constant  Value=motor_num
  Demux : Demux  Outputs=3
  Demux1 : Demux  Outputs=3
  Demux2 : Demux  Outputs=3
  Divide : Product  Inputs=*/
  Gain : Gain  Gain=R_rotor
  Gain1 : Gain  Gain=[-1 0 1]
  Gain2 : Gain  Gain=1/2*rho*(R_rotor^2*pi)
  Gain3 : Gain  Gain=-1
  Gain4 : Gain  Gain=-1
  Gain5 : Gain  Gain=R_rotor
  Gain6 : Gain  Gain=R_rotor
  MATLAB Function : MATLAB Function  TreatAsAtomicUnit=on
  Mux : Mux
  Product1 : Product
  Product2 : Product  Multiplication=Matrix(*)
  Product3 : Product
  Product4 : Product  Multiplication=Matrix(*)
  Selector : Selector  InputPortWidth=4  IndexOptions=Index vector (port)  Indices=[1 3]  OutputSizes=1
  Selector1 : Selector  InputPortWidth=4  IndexOptions=Index vector (port)  Indices=[1 3]  OutputSizes=1
  Selector2 : Selector  NumberOfDimensions=3  InputPortWidth=4  IndexOptions=Select all,Select all,Index vector (port)  Indices=[1 3],1,1  OutputSizes=1,1,1
  Square : Math  Operator=square  SaturateOnIntegerOverflow=on
  Terminator : Terminator
  forces (wind frame) : Gain  Gain=[0 -1 0 0 ; 0 0 0 0 ; -1 0 0 0]  Multiplication=Matrix(K*u) (u vector)
  moments (wind frame) : Gain  Gain=[0 0 0 -1 ; 0 0 0 0 ; 0 0 1 0]  Multiplication=Matrix(K*u) (u vector)
  H : Outport
  Y : Outport  Port=2
  T : Outport  Port=3
  Mx : Outport  Port=4
  My : Outport  Port=5
  Q : Outport  Port=6
  wires:
  Demux/2 -> Terminator/1
  Mux/1 -> Product3/1
  Selector2/1 -> MATLAB Function/2(R_BR)
  Gain4/1 -> T/1
  Demux1/3 -> Gain4/1
  Demux/3 -> "C_T "/2, C_H/2, C_Q/2, C_M/2
  Constant2/1 -> Selector/2, Selector1/2, Selector2/2
  Selector/1 -> Gain/1
  Gain2/1 -> Product3/2  "mu"
  Constant1/1 -> Selector2/1
  Demux1/1 -> Gain3/1
  "C_T "/1 -> Mux/1
  Product4/1 -> Demux2/1
  moments (wind frame)/1 -> Product4/2
  Divide/1 -> Gain1/1
  Square/1 -> Gain2/1
  Demux/1 -> "C_T "/1, C_H/1, C_Q/1, C_M/1
  C_M/1 -> Product1/1
  C_H/1 -> Mux/2
  Product2/1 -> Demux1/1
  Demux1/2 -> Y/1
  omega/1 -> Selector/1
  Demux2/3 -> Q/1
  vB/1 -> MATLAB Function/1(vB)
  MATLAB Function/1(R_RW) -> Product2/1, Product4/1
  Selector1/1 -> Product1/2
  Demux2/1 -> Mx/1
  MATLAB Function/2(vW) -> Divide/1
  Gain1/1 -> Demux/1  "mu"
  Product3/1 -> moments (wind frame)/1, forces (wind frame)/1
  forces (wind frame)/1 -> Product2/2
  Gain/1 -> Divide/2, Square/1  "VT"
  Demux2/2 -> My/1
  Constant/1 -> Selector1/1
  Gain3/1 -> H/1
  Gain6/1 -> Mux/4
  Gain5/1 -> Mux/3
  Product1/1 -> Gain6/1
  C_Q/1 -> Gain5/1

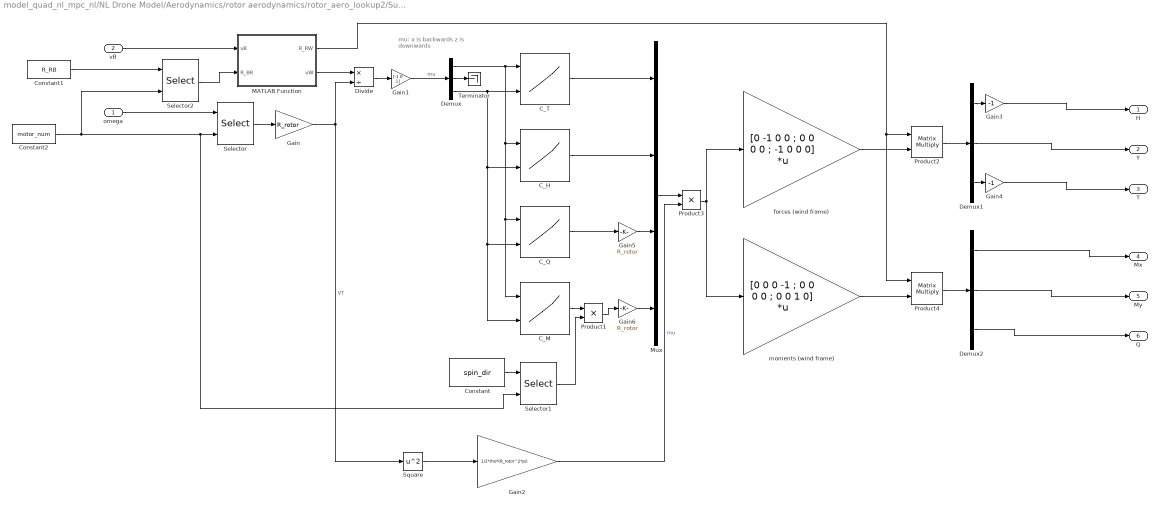
== system model_quad_nl_mpc_nl/NL Drone Model/Aerodynamics/rotor aerodynamics/rotor_aero_lookup2/Subsystem3 ==
  note: mu:
      | x is backwards
      | z is downwards
  omega : Inport
  vB : Inport  Port=2
  C_H : Lookup_n-D  BreakpointsForDimension1=rotorAero.mu_x_loops  BreakpointsForDimension2=rotorAero.mu_z_loops  Table=rotorAero.C_H  InternalRulePriority=Speed  RndMeth=Simplest  InputSameDT=on
      settings: InputPortMap=u0,u1
  C_M : Lookup_n-D  BreakpointsForDimension1=rotorAero.mu_x_loops  BreakpointsForDimension2=rotorAero.mu_z_loops  Table=rotorAero.C_M  InternalRulePriority=Speed  RndMeth=Simplest  InputSameDT=on
      settings: InputPortMap=u0,u1
  C_Q : Lookup_n-D  BreakpointsForDimension1=rotorAero.mu_x_loops  BreakpointsForDimension2=rotorAero.mu_z_loops  Table=rotorAero.C_Q  InternalRulePriority=Speed  RndMeth=Simplest  InputSameDT=on
      settings: InputPortMap=u0,u1
  "C_T " : Lookup_n-D  BreakpointsForDimension1=rotorAero.mu_x_loops  BreakpointsForDimension2=rotorAero.mu_z_loops  Table=rotorAero.C_T  InternalRulePriority=Speed  RndMeth=Simplest  InputSameDT=on
      settings: InputPortMap=u0,u1
  Constant : Constant  Value=spin_dir
  Constant1 : Constant  Value=R_RB
  Constant2 : Constant  Value=motor_num
  Demux : Demux  Outputs=3
  Demux1 : Demux  Outputs=3
  Demux2 : Demux  Outputs=3
  Divide : Product  Inputs=*/
  Gain : Gain  Gain=R_rotor
  Gain1 : Gain  Gain=[-1 0 1]
  Gain2 : Gain  Gain=1/2*rho*(R_rotor^2*pi)
  Gain3 : Gain  Gain=-1
  Gain4 : Gain  Gain=-1
  Gain5 : Gain  Gain=R_rotor
  Gain6 : Gain  Gain=R_rotor
  MATLAB Function : MATLAB Function  TreatAsAtomicUnit=on
  Mux : Mux
  Product1 : Product
  Product2 : Product  Multiplication=Matrix(*)
  Product3 : Product
  Product4 : Product  Multiplication=Matrix(*)
  Selector : Selector  InputPortWidth=4  IndexOptions=Index vector (port)  Indices=[1 3]  OutputSizes=1
  Selector1 : Selector  InputPortWidth=4  IndexOptions=Index vector (port)  Indices=[1 3]  OutputSizes=1
  Selector2 : Selector  NumberOfDimensions=3  InputPortWidth=4  IndexOptions=Select all,Select all,Index vector (port)  Indices=[1 3],1,1  OutputSizes=1,1,1
  Square : Math  Operator=square  SaturateOnIntegerOverflow=on
  Terminator : Terminator
  forces (wind frame) : Gain  Gain=[0 -1 0 0 ; 0 0 0 0 ; -1 0 0 0]  Multiplication=Matrix(K*u) (u vector)
  moments (wind frame) : Gain  Gain=[0 0 0 -1 ; 0 0 0 0 ; 0 0 1 0]  Multiplication=Matrix(K*u) (u vector)
  H : Outport
  Y : Outport  Port=2
  T : Outport  Port=3
  Mx : Outport  Port=4
  My : Outport  Port=5
  Q : Outport  Port=6
  wires:
  C_Q/1 -> Gain5/1
  Product1/1 -> Gain6/1
  Gain5/1 -> Mux/3
  Gain6/1 -> Mux/4
  Gain3/1 -> H/1
  Constant/1 -> Selector1/1
  Demux2/2 -> My/1
  Gain/1 -> Square/1, Divide/2  "VT"
  forces (wind frame)/1 -> Product2/2
  Product3/1 -> forces (wind frame)/1, moments (wind frame)/1
  Gain1/1 -> Demux/1  "mu"
  MATLAB Function/2(vW) -> Divide/1
  Demux2/1 -> Mx/1
  Selector1/1 -> Product1/2
  MATLAB Function/1(R_RW) -> Product4/1, Product2/1
  vB/1 -> MATLAB Function/1(vB)
  Demux2/3 -> Q/1
  omega/1 -> Selector/1
  Demux1/2 -> Y/1
  Product2/1 -> Demux1/1
  C_H/1 -> Mux/2
  C_M/1 -> Product1/1
  Demux/1 -> C_M/1, C_Q/1, C_H/1, "C_T "/1
  Square/1 -> Gain2/1
  Divide/1 -> Gain1/1
  moments (wind frame)/1 -> Product4/2
  Product4/1 -> Demux2/1
  "C_T "/1 -> Mux/1
  Demux1/1 -> Gain3/1
  Constant1/1 -> Selector2/1
  Gain2/1 -> Product3/2  "mu"
  Selector/1 -> Gain/1
  Constant2/1 -> Selector2/2, Selector1/2, Selector/2
  Demux/3 -> C_M/2, C_Q/2, C_H/2, "C_T "/2
  Demux1/3 -> Gain4/1
  Gain4/1 -> T/1
  Selector2/1 -> MATLAB Function/2(R_BR)
  Mux/1 -> Product3/1
  Demux/2 -> Terminator/1

== matlab function model_quad_nl_mpc_nl/MATLAB Function ==
  data: x input; y output; ref input
function y = fcn(x,ref)

y = zeros(1,2);
y(1) = x(3);
y(2) = ref(9);

end

== matlab function model_quad_nl_mpc_nl/NL Drone Model/Aerodynamics/rotor aerodynamics/rotor_aero_lookup2/Subsystem2/MATLAB Function ==
  data: vB input; R_RW output; R_BR input; vW output
function [R_RW,vW] = toXZplane(vB,R_BR)
% vB is vehicle velocity vector in body coords (IAS - i.e. relative to
% local air; wind must be inverted)
% R_BRa is rotation matrix from body frame to rotor frame (z along shaft, x
% usually forwards)
% R_RW is rotation matrix from rotor frame to wind frame (z aligned with
% shaft, wind aligned with xz plane)
% vW is the 3 element wind vector transformed by R_RW.' to lie in the "wind
% frame" where only the 1st and 3rd elements can be nonzero.

% define output sizes
R_RW = zeros(3,3);
vW   = zeros(3,1);

% convert vehicle velocity in body frame to relative wind velocity in rotor frame
vR = -R_BR.'*vB(:);

% determine transform to align rotor XZ plane with relative wind (R is
% nominal rotor frame, W is rotated about z to align wind in XZ plane)
if vR(1)==0 && vR(2)==0, % wind is zero or aligned with Z axis
    R_RW = eye(3);
else
    h = (vR(1)^2 + vR(2)^2)^0.5; % size of vR projected on XY plane (NB this is mu_x component)
    %a = atan2(vW(2),vW(1)) 
    c = vR(1)/h; %cos(a); 
    s = vR(2)/h; %sin(a);
    R_RW = [ c -s 0 ; s c 0 ; 0 0 1];
end

% get relative wind in XZ plane
vW = R_RW.' * vR;

== matlab function model_quad_nl_mpc_nl/NL Drone Model/Aerodynamics/rotor aerodynamics/rotor_aero_lookup2/Subsystem3/MATLAB Function ==
  data: vB input; R_RW output; R_BR input; vW output
function [R_RW,vW] = toXZplane(vB,R_BR)
% vB is vehicle velocity vector in body coords (IAS - i.e. relative to
% local air; wind must be inverted)
% R_BRa is rotation matrix from body frame to rotor frame (z along shaft, x
% usually forwards)
% R_RW is rotation matrix from rotor frame to wind frame (z aligned with
% shaft, wind aligned with xz plane)
% vW is the 3 element wind vector transformed by R_RW.' to lie in the "wind
% frame" where only the 1st and 3rd elements can be nonzero.

% define output sizes
R_RW = zeros(3,3);
vW   = zeros(3,1);

% convert vehicle velocity in body frame to relative wind velocity in rotor frame
vR = -R_BR.'*vB(:);

% determine transform to align rotor XZ plane with relative wind (R is
% nominal rotor frame, W is rotated about z to align wind in XZ plane)
if vR(1)==0 && vR(2)==0, % wind is zero or aligned with Z axis
    R_RW = eye(3);
else
    h = (vR(1)^2 + vR(2)^2)^0.5; % size of vR projected on XY plane (NB this is mu_x component)
    %a = atan2(vW(2),vW(1)) 
    c = vR(1)/h; %cos(a); 
    s = vR(2)/h; %sin(a);
    R_RW = [ c -s 0 ; s c 0 ; 0 0 1];
end

% get relative wind in XZ plane
vW = R_RW.' * vR;
